simulink model "WGmodel_v7"  (R2022b)
settings: Solver=VariableStepAuto  StartTime=0.0  StopTime=100  RelTol=1e-3
values from neighbouring files (symbols this model uses):
  m_pw = zeros(nvw,nwr)    [fun_getwindpowercurve_v4.m]
  pinitwindgen = 0.5161    [WGmodel_startup.m]    (also in WGmodel_startup_v2.m; WGmodel_startup_v3.m = pinitwindgen(1))
  R = 0.05    [WGmodel_startup.m]    (also in WGmodel_startup_v2.m; WGmodel_startup_v3.m)
  Tc1 = 0.05    [WGmodel_startup.m]    (also in WGmodel_startup_v2.m; WGmodel_startup_v3.m)
  Tc2 = 0.05    [WGmodel_startup.m]    (also in WGmodel_startup_v2.m; WGmodel_startup_v3.m)
  v_beta = 0:1:2    [WGmodel_startup.m]    (also in fun_getwindpowercurve_v2.m = 0.5)
  v_pwdel = 0.9 * max(m_pw,[],2)    [fun_getwindpowercurve_v2.m]    (also in fun_getwindpowercurve_v3.m = (1-deload) * v_pwmpp; fun_getwindpowercurve_v4.m = (1-deload) * v_pwmpp)
  v_pwmpp = zeros(nvw,1)    [fun_getwindpowercurve_v4.m]
  v_vw = 5:10    [LUT_2D.m]    (also in WGmodel_startup.m = 5:1:10; WGmodel_startup_v2.m = 5:1:15; WGmodel_startup_v3.m = 5:.5:12; fun_getwindpowercurve_v2.m = [10 11 12])
  v_wr = v_Wr/Wrn    [fun_getwindpowercurve.m]    (also in fun_getwindpowercurve_v2.m; fun_getwindpowercurve_v3.m; fun_getwindpowercurve_v4.m; fun_getwindpowercurve_v5.m)
  v_wrdel = (v_wr(v_iwrmpp+i_lower)+v_wr(v_iwrmpp+i_higher))/2    [fun_getwindpowercurve_v2.m]    (also in fun_getwindpowercurve_v3.m = v_Wrdel/Wrn; fun_getwindpowercurve_v4.m = v_Wrdel/Wrn)
  v_wrmpp = v_Wrmpp/Wrn    [fun_getwindpowercurve.m]    (also in fun_getwindpowercurve_v2.m; fun_getwindpowercurve_v3.m; fun_getwindpowercurve_v4.m)
  wr0 = wr0(1)    [WGmodel_startup_v3.m]
libraries: simulink x1
settings Model: Creator=User  LastModifiedBy=User

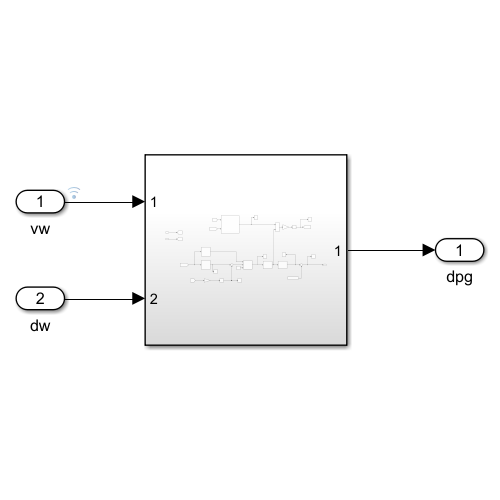
[thumbnail: Simulink's stored preview of the top-level diagram]
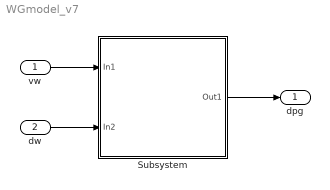
== system WGmodel_v7 ==
  vw : Inport
  dw : Inport  Port=2
  Subsystem : Subsystem
  dpg : Outport
  wires:
  vw/1 -> Subsystem/1(In1)
  dw/1 -> Subsystem/2(In2)
  Subsystem/1(Out1) -> dpg/1

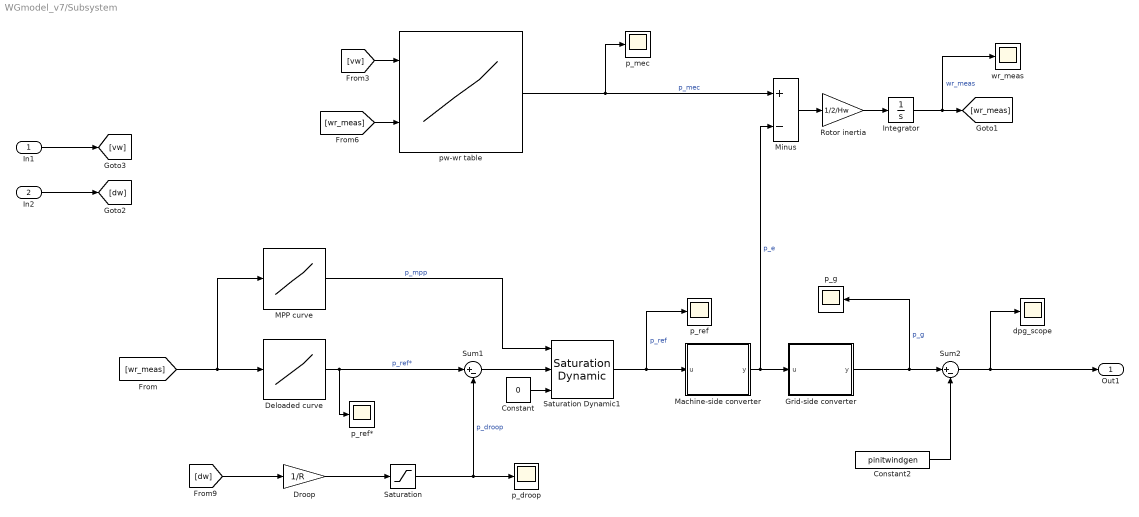
== system WGmodel_v7/Subsystem ==
  In1 : Inport
  In2 : Inport  Port=2
  Constant : Constant  Value=0
  Constant2 : Constant  Value=pinitwindgen
  Deloaded curve : Lookup_n-D  NumberOfTableDimensions=1  BreakpointsForDimension1=v_wrdel  Table=v_pwdel  InternalRulePriority=Speed  RndMeth=Simplest
  Droop : Gain  Gain=1/R
  Grid-side converter : Subsystem  mask{T=Tc2, y0=pinitwindgen}
      mask prompts: T "Time constant (s)"; y0 "Initial condition (pu)"
  Integrator : Integrator  InitialCondition=wr0
  MPP curve : Lookup_n-D  NumberOfTableDimensions=1  BreakpointsForDimension1=v_wrmpp  Table=v_pwmpp  InternalRulePriority=Speed  RndMeth=Simplest
  Machine-side converter : Subsystem  mask{T=Tc1, y0=pinitwindgen}
      mask prompts: T "Time constant (s)"; y0 "Initial condition (pu)"
  Minus : Sum  Inputs=+-
  Rotor inertia : Gain  Gain=1/2/Hw
  Saturation : Saturate  UpperLimit=v_pwdel(length(v_pwdel))  LowerLimit=-v_pwdel(length(v_pwdel))
  Saturation Dynamic1 : simulink/Discontinuities/Saturation Dynamic  OutMin=0  OutMax=[]  OutDataTypeStr=Inherit: Same as second input  OutDataType=fixdt(1, 16)  OutScaling=2^-10  DoSatur=off
  Sum1 : Sum  Inputs=|+-
  Sum2 : Sum  Inputs=|+-
  dpg_scope : Scope
  p_droop : Scope
  p_g : Scope
  p_mec : Scope
  p_ref : Scope
  p_ref* : Scope
  pw-wr table : Lookup_n-D  BreakpointsForDimension1=v_vw  BreakpointsForDimension2=v_wr  BreakpointsForDimension3=v_beta  Table=m_pw  InternalRulePriority=Speed  RndMeth=Simplest
      settings: InputPortMap=u0,u1
  wr_meas : Scope
  Out1 : Outport
  wires:
  Sum2/1 -> Out1/1, dpg_scope/1
  [wr_meas] -> pw-wr table/2
  Deloaded curve/1 -> Sum1/1, p_ref*/1  "p_ref*"
  [dw] -> Droop/1
  Grid-side converter/1(y) -> Sum2/1, p_g/1  "p_g"
  Saturation Dynamic1/1 -> p_ref/1, Machine-side converter/1(u)  "p_ref"
  [wr_meas] -> Deloaded curve/1, MPP curve/1
  Saturation/1 -> p_droop/1, Sum1/2  "p_droop"
  Rotor inertia/1 -> Integrator/1
  [vw] -> pw-wr table/1
  pw-wr table/1 -> Minus/1, p_mec/1  "p_mec"
  Minus/1 -> Rotor inertia/1
  Integrator/1 -> wr_meas/1, [wr_meas]  "wr_meas"
  In1/1 -> [vw]
  Sum1/1 -> Saturation Dynamic1/2
  Machine-side converter/1(y) -> Minus/2, Grid-side converter/1(u)  "p_e"
  Droop/1 -> Saturation/1
  MPP curve/1 -> Saturation Dynamic1/1  "p_mpp"
  Constant2/1 -> Sum2/2
  In2/1 -> [dw]
  Constant/1 -> Saturation Dynamic1/3

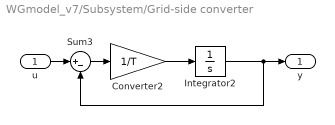
== system WGmodel_v7/Subsystem/Grid-side converter ==
  u : Inport
  Converter2 : Gain  Gain=1/T
  Integrator2 : Integrator  InitialCondition=y0
  Sum3 : Sum  Inputs=|+-
  y : Outport
  wires:
  Integrator2/1 -> y/1, Sum3/2
  Sum3/1 -> Converter2/1
  Converter2/1 -> Integrator2/1
  u/1 -> Sum3/1

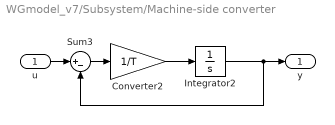
== system WGmodel_v7/Subsystem/Machine-side converter ==
  u : Inport
  Converter2 : Gain  Gain=1/T
  Integrator2 : Integrator  InitialCondition=y0
  Sum3 : Sum  Inputs=|+-
  y : Outport
  wires:
  Integrator2/1 -> y/1, Sum3/2
  Sum3/1 -> Converter2/1
  Converter2/1 -> Integrator2/1
  u/1 -> Sum3/1
